simulink model "Nonlinear_withSMC_Final"  (R2022b)
settings: Solver=VariableStepAuto  StartTime=0.0  StopTime=80  RelTol=1e-3
values from neighbouring files (symbols this model uses):
  Lcont = -inv(Sreg*Breg)*((Sreg*Areg)-(Phi*Sreg))*Tr    [Sliding_surface_design.m]
  S = [Mc eye(mm)]*Tr    [Sliding_surface_design.m]
  x1 = X1.Data(:,1)    [Ploting.m]
undefined symbols (not defined in the file or in its folder): u1
settings Model: Creator=henrr  LastModifiedBy=henrr
settings DataIOCC: SaveOutput=off  SaveTime=off  ReturnWorkspaceOutputs=off

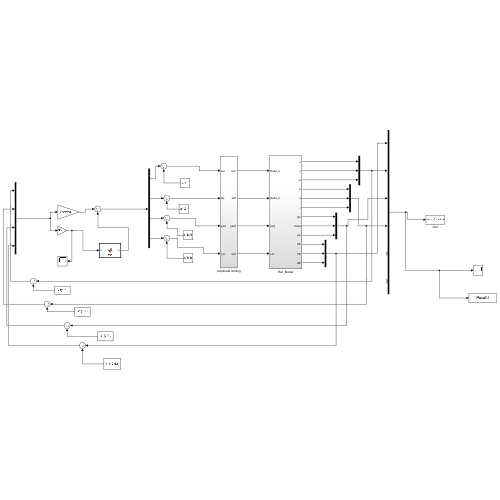
[thumbnail: Simulink's stored preview of the top-level diagram]
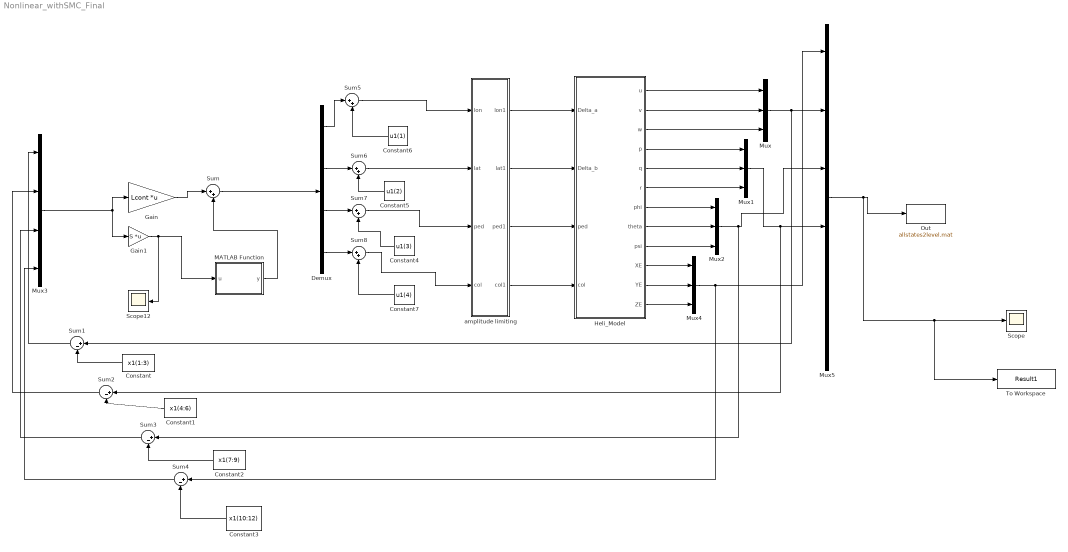
== system Nonlinear_withSMC_Final ==
  Constant : Constant  Value=x1(1:3)
  Constant1 : Constant  Value=x1(4:6)
  Constant2 : Constant  Value=x1(7:9)
  Constant3 : Constant  Value=x1(10:12)
  Constant4 : Constant  Value=u1(3)
  Constant5 : Constant  Value=u1(2)
  Constant6 : Constant  Value=u1(1)
  Constant7 : Constant  Value=u1(4)
  Demux : Demux
  Gain : Gain  Gain=Lcont  Multiplication=Matrix(K*u)
  Gain1 : Gain  Gain=S  Multiplication=Matrix(K*u)
  Heli_Model : Subsystem
  MATLAB Function : MATLAB Function  TreatAsAtomicUnit=on
  Mux{,1..2,4} (4 alike) : Mux  Inputs=3
  Mux3 : Mux
  Mux5 : Mux  Inputs=6
  Out : ToFile  Filename=allstates2level.mat  MatrixName=AllStates
  Scope : Scope
  Scope12 : Scope
  Sum{,5..8} (5 alike) : Sum  Inputs=|++
  Sum{1..4} (4 alike) : Sum  Inputs=|+-
  To Workspace : ToWorkspace  VariableName=Result1  SaveFormat=Timeseries  SampleTime=-1
  amplitude limiting : Subsystem
  wires:
  Heli_Model/12(ZE) -> Mux4/3
  amplitude limiting/4(col1) -> Heli_Model/4(col)
  Heli_Model/9(psi) -> Mux2/3
  amplitude limiting/1(lon1) -> Heli_Model/1(Delta_a)
  Heli_Model/2(v) -> Mux/2
  Mux/1 -> Sum1/1, Mux5/2
  Heli_Model/6(r) -> Mux1/3
  Heli_Model/1(u) -> Mux/1
  Mux5/1 -> To Workspace/1, Scope/1, Out/1
  Mux2/1 -> Sum3/1, Mux5/3
  Heli_Model/11(YE) -> Mux4/2
  Mux1/1 -> Sum2/1, Mux5/4
  Heli_Model/8(theta) -> Mux2/2
  Heli_Model/4(p) -> Mux1/1
  Heli_Model/3(w) -> Mux/3
  Mux4/1 -> Sum4/1, Mux5/1
  Heli_Model/5(q) -> Mux1/2
  amplitude limiting/3(ped1) -> Heli_Model/3(ped)
  Heli_Model/10(XE) -> Mux4/1
  amplitude limiting/2(lat1) -> Heli_Model/2(Delta_b)
  Heli_Model/7(phi) -> Mux2/1
  Gain1/1 -> Scope12/1, MATLAB Function/1(u)
  Sum/1 -> Demux/1
  Gain/1 -> Sum/1
  Mux3/1 -> Gain1/1, Gain/1
  MATLAB Function/1(y) -> Sum/2
  Sum1/1 -> Mux3/1
  Sum2/1 -> Mux3/2
  Sum3/1 -> Mux3/3
  Sum4/1 -> Mux3/4
  Constant/1 -> Sum1/2
  Constant1/1 -> Sum2/2
  Constant2/1 -> Sum3/2
  Constant3/1 -> Sum4/2
  Sum5/1 -> amplitude limiting/1(lon)
  Sum6/1 -> amplitude limiting/2(lat)
  Sum7/1 -> amplitude limiting/3(ped)
  Sum8/1 -> amplitude limiting/4(col)
  Demux/1 -> Sum5/1
  Demux/2 -> Sum6/1
  Demux/3 -> Sum7/1
  Demux/4 -> Sum8/1
  Constant6/1 -> Sum5/2
  Constant5/1 -> Sum6/2
  Constant4/1 -> Sum7/2
  Constant7/1 -> Sum8/2

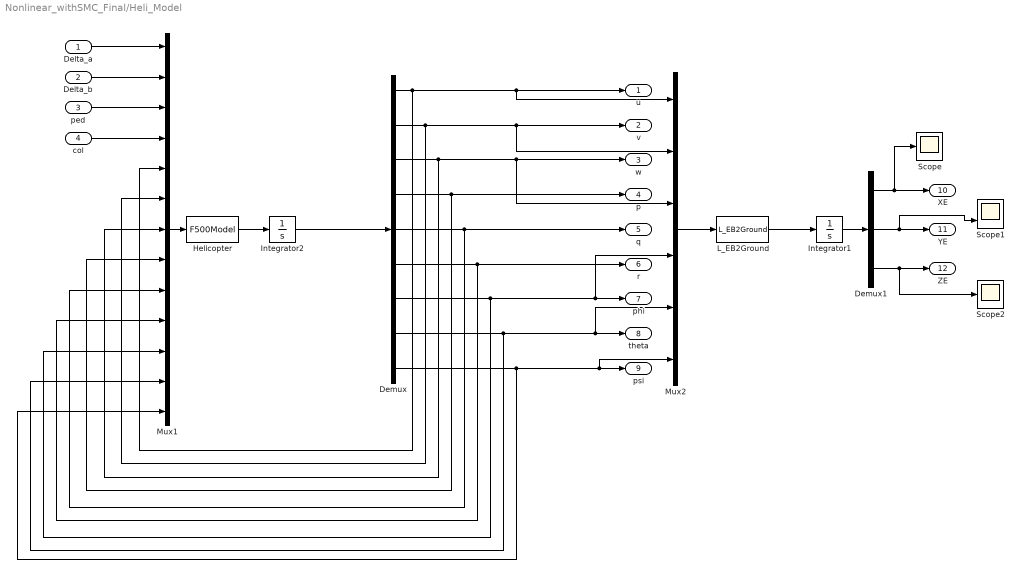
== system Nonlinear_withSMC_Final/Heli_Model ==
  Delta_a : Inport
  Delta_b : Inport  Port=2
  ped : Inport  Port=3
  col : Inport  Port=4
  Demux : Demux  Outputs=9
  Demux1 : Demux  Outputs=3
  Helicopter : MATLABFcn  MATLABFcn=F500Model
  Integrator1 : Integrator  InitialCondition=[0 0 0]
  Integrator2 : Integrator  InitialCondition=[0 0 0 0 0 0 0 0 0]
  L_EB2Ground : MATLABFcn  MATLABFcn=L_EB2Ground
  Mux1 : Mux  Inputs=13
  Mux2 : Mux  Inputs=6
  Scope : Scope
  Scope1 : Scope  NumInputPorts=2
  Scope2 : Scope
  u : Outport
  v : Outport  Port=2
  w : Outport  Port=3
  p : Outport  Port=4
  q : Outport  Port=5
  r : Outport  Port=6
  phi : Outport  Port=7
  theta : Outport  Port=8
  psi : Outport  Port=9
  XE : Outport  Port=10
  YE : Outport  Port=11
  ZE : Outport  Port=12
  wires:
  Demux/1 -> Mux1/5, u/1, Mux2/1
  Demux/2 -> Mux1/6, v/1, Mux2/2
  Demux/3 -> Mux1/7, w/1, Mux2/3
  Demux/4 -> Mux1/8, p/1
  Demux/5 -> Mux1/9, q/1
  Demux/6 -> Mux1/10, r/1
  Demux/7 -> Mux1/11, phi/1, Mux2/4
  Demux/8 -> Mux1/12, theta/1, Mux2/5
  Demux/9 -> Mux1/13, psi/1, Mux2/6
  Demux1/1 -> XE/1, Scope/1
  Demux1/2 -> YE/1, Scope1/2
  Demux1/3 -> ZE/1, Scope2/1
  Mux2/1 -> L_EB2Ground/1
  L_EB2Ground/1 -> Integrator1/1
  Integrator1/1 -> Demux1/1
  Mux1/1 -> Helicopter/1
  col/1 -> Mux1/4
  Integrator2/1 -> Demux/1
  ped/1 -> Mux1/3
  Delta_a/1 -> Mux1/1
  Delta_b/1 -> Mux1/2
  Helicopter/1 -> Integrator2/1

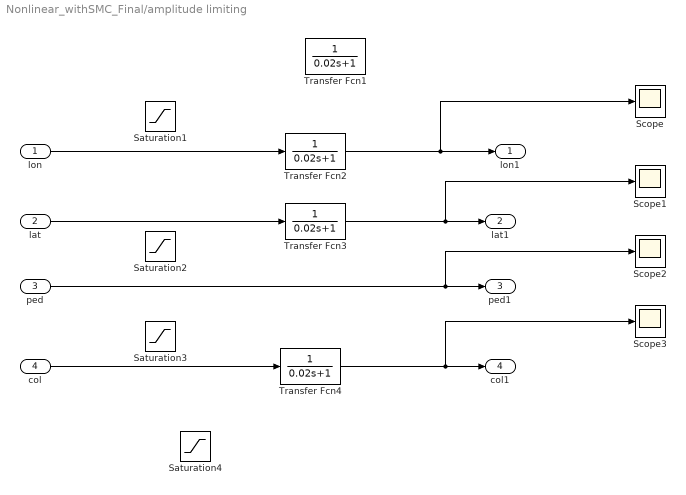
== system Nonlinear_withSMC_Final/amplitude limiting ==
  lon : Inport
  lat : Inport  Port=2
  ped : Inport  Port=3
  col : Inport  Port=4
  Saturation1 : Saturate  UpperLimit=0.6  LowerLimit=-0.6
  Saturation2 : Saturate  UpperLimit=0.6  LowerLimit=-0.6
  Saturation3 : Saturate  UpperLimit=0.6  LowerLimit=-0.6
  Saturation4 : Saturate  UpperLimit=10  LowerLimit=-10
  Scope{,1..3} (4 alike) : Scope
  Transfer Fcn{1..4} (4 alike) : TransferFcn  Denominator=[0.02 1]
  lon1 : Outport
  lat1 : Outport  Port=2
  ped1 : Outport  Port=3
  col1 : Outport  Port=4
  wires:
  lon/1 -> Transfer Fcn2/1
  lat/1 -> Transfer Fcn3/1
  col/1 -> Transfer Fcn4/1
  ped/1 -> ped1/1, Scope2/1
  Transfer Fcn2/1 -> lon1/1, Scope/1
  Transfer Fcn3/1 -> lat1/1, Scope1/1
  Transfer Fcn4/1 -> col1/1, Scope3/1

== matlab function Nonlinear_withSMC_Final/MATLAB Function ==
  data: u input; y output
function y = fcn(u)

 Lam=[11.5782    0.0000   -0.0000   -0.0000;
   -0.0000  -12.2181    0.0000   -0.0000;
    0.0000   -0.0000    0.6730    0.6449;
    0.0000   -0.0000   -0.0000   -0.4301];

P = [0.0250         0         0         0;
         0    0.0250         0         0;
         0         0    0.0250         0;
         0         0         0    0.0250;];

y = -10*inv(Lam)*P*u/(norm(P*u)+0.001);
